simulink model "Modulary_loads"  (Simulink 8.1)
settings: Solver=ode23t  StartTime=0.0  StopTime=tfin  RelTol=1e-3
values from neighbouring files (symbols this model uses):
  C = 0    [Sketch_controller_model_ini.m]    (also in Symmetry_REAL_TIME_ini.m = 0.005; Symmetry_ini_Modulary.m = 0.02)
  C_ref = 20e-3    (= 0.02)    [Symmetry_ini_Modulary.m]
  IO = [1,1,1]    [Symmetry_ini_Modulary.m]
  main_IO = 1    [Symmetry_ini_Modulary.m]
  R = 100    [Sketch_controller_model_ini.m]    (also in Symmetry_REAL_TIME_ini.m; Symmetry_ini_Modulary.m = 50)
  R_ref = 50    [Symmetry_ini_Modulary.m]
  sample = 10e-5    (= 0.0001)    [Inverter_ini.m]    (also in Sketch_controller_model_ini.m; Symmetry_REAL_TIME_ini.m; Symmetry_ini.m; Symmetry_ini_COPY.m)
libraries: powerlib x17, powerlib_extras x3
settings Model: Creator=Neukirchner László  LastModifiedBy=Neukirchner László
settings SolverCC: ZeroCrossAlgorithm=Adaptive  SolverResetMethod=Robust
settings DataIOCC: SignalLoggingSaveFormat=Dataset
settings OptimizationCC: ExpressionDepthLimit=128
settings DebuggingCC: FcnCallInpInsideContextMsg=EnableAllAsError
settings GRTTargetCC: CombineOutputUpdateFcns=on  GRTInterface=off

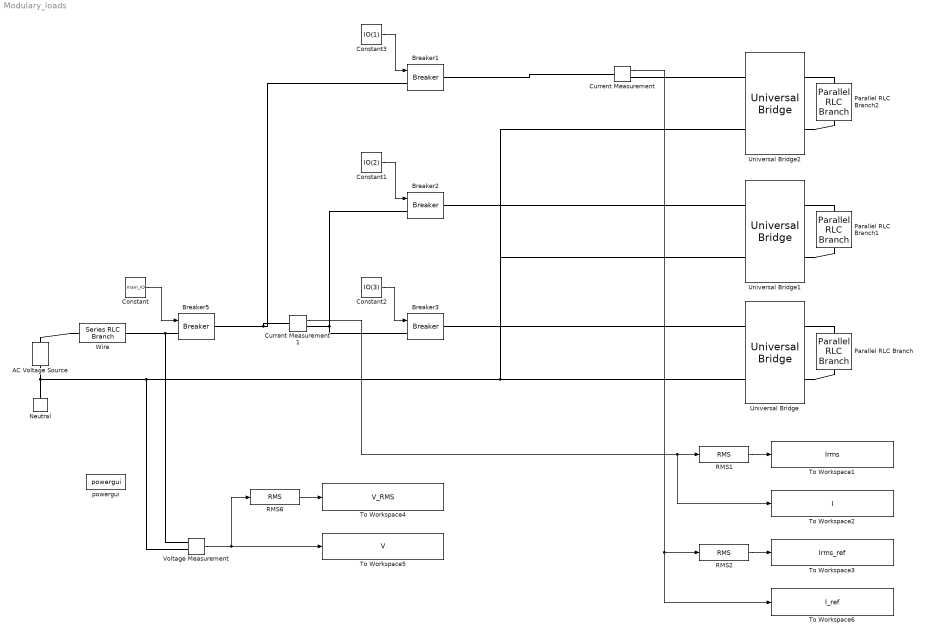
== system Modulary_loads ==
  AC Voltage Source : powerlib/Electrical Sources/AC Voltage Source  Amplitude=230*sqrt(2)  Phase=0  Frequency=50  SampleTime=sample  Measurements=None
  Breaker{1..3,5} (4 alike) : powerlib/Elements/Breaker  BreakerResistance=0.01  InitialState=0  SnubberResistance=1e7  SnubberCapacitance=inf  SwitchingTimes="[ 1/60  5/60 ]"  External=on  Measurements=None  MoreParameters=off  NoBreakLoop=off
  Constant : Constant  Value=main_IO
  Constant1 : Constant  Value=IO(2)
  Constant2 : Constant  Value=IO(3)
  Constant3 : Constant  Value=IO(1)
  Current Measurement : powerlib/Measurements/Current Measurement  PhasorSimulation=off  OutputType=Complex  PSBequivalent=0
  Current Measurement1 : powerlib/Measurements/Current Measurement  PhasorSimulation=off  OutputType=Complex  PSBequivalent=0
  Neutral : powerlib/Elements/Neutral  LConnTagsString=a  NodeNumber=10
  Parallel RLC Branch : powerlib/Elements/Parallel RLC Branch  LConnTagsString=a  RConnTagsString=__new0  BranchType=RC  Resistance=R  Inductance=1e-3  SetiL0=off  InitialCurrent=0  Capacitance=C  Setx0=off  InitialVoltage=0  Measurements=None
  Parallel RLC Branch1 : powerlib/Elements/Parallel RLC Branch  LConnTagsString=a  RConnTagsString=__new0  BranchType=RC  Resistance=R  Inductance=1e-3  SetiL0=off  InitialCurrent=0  Capacitance=C  Setx0=off  InitialVoltage=0  Measurements=None
  Parallel RLC Branch2 : powerlib/Elements/Parallel RLC Branch  LConnTagsString=a  RConnTagsString=__new0  BranchType=RC  Resistance=R_ref  Inductance=1e-3  SetiL0=off  InitialCurrent=0  Capacitance=C_ref  Setx0=off  InitialVoltage=0  Measurements=None
  RMS1 : powerlib_extras/Measurements/RMS  f1=50
  RMS2 : powerlib_extras/Measurements/RMS  f1=50
  RMS6 : powerlib_extras/Measurements/RMS  f1=50
  To Workspace1 : ToWorkspace  VariableName=Irms  SampleTime=sample  SaveFormat=Timeseries
  To Workspace2 : ToWorkspace  VariableName=I  SampleTime=sample  SaveFormat=Timeseries
  To Workspace3 : ToWorkspace  VariableName=Irms_ref  SampleTime=sample  SaveFormat=Timeseries
  To Workspace4 : ToWorkspace  VariableName=V_RMS  SampleTime=sample  SaveFormat=Timeseries
  To Workspace5 : ToWorkspace  VariableName=V  SampleTime=sample  SaveFormat=Timeseries
  To Workspace6 : ToWorkspace  VariableName=I_ref  SampleTime=sample  SaveFormat=Timeseries
  Universal Bridge : powerlib/Power Electronics/Universal Bridge  Arms=2  SnubberResistance=1e5  SnubberCapacitance=inf  Device=Diodes  Ron=1e-3  Lon=0  ForwardVoltages="[  0  0  ]"  ForwardVoltage=0.8  GTOparameters=[ 10e-6 , 20e-6 ]  IGBTparameters=[ 1e-6 , 2e-6 ]  Measurements=None  Measurements_2=None  converterType=Rectifier
  Universal Bridge1 : powerlib/Power Electronics/Universal Bridge  Arms=2  SnubberResistance=1e5  SnubberCapacitance=inf  Device=Diodes  Ron=1e-3  Lon=0  ForwardVoltages="[  0  0  ]"  ForwardVoltage=0.8  GTOparameters=[ 10e-6 , 20e-6 ]  IGBTparameters=[ 1e-6 , 2e-6 ]  Measurements=None  Measurements_2=None  converterType=Rectifier
  Universal Bridge2 : powerlib/Power Electronics/Universal Bridge  Arms=2  SnubberResistance=1e5  SnubberCapacitance=inf  Device=Diodes  Ron=1e-3  Lon=0  ForwardVoltages="[  0  0  ]"  ForwardVoltage=0.8  GTOparameters=[ 10e-6 , 20e-6 ]  IGBTparameters=[ 1e-6 , 2e-6 ]  Measurements=None  Measurements_2=None  converterType=Rectifier
  Voltage Measurement : powerlib/Measurements/Voltage Measurement  PhasorSimulation=off  OutputType=Complex  PSBequivalent=0
  Wire : powerlib/Elements/Series RLC Branch  LConnTagsString=__new0  RConnTagsString=__new0  BranchType=RL  Resistance=0.4  Inductance=1e-3  SetiL0=off  InitialCurrent=0  Capacitance=1e-6  Setx0=off  InitialVoltage=0  Measurements=None
  powergui : powerlib/powergui  SimulationMode=Continuous  SolverType=Tustin  SampleTime=50e-6  frequency=60  SPID=off  DisableSnubberDevices=off  DisableRonSwitches=off  DisableVfSwitches=off  SwTol=0  Interpol=off  DisplayEquations=off  frequencyindice=0  Pbase=100e6  ErrMax=1e-4  Iterations=50  UnitsV=kV  UnitsW=MW  FunctionMessages=off  echomessages=off  HookPort=off  EnableUseOfTLC=off  x0status=blocks  RestoreLinks=warning  ResistiveCurrentMeasurement=off  Frange=[0:2:500]  Ylog=off  Xlog=on  ShowGrid=off  save=off  variable=ZData  structure=0  ZoomFFT=on  StartTime=0.0  cycles=1  DisplayStyle=1  fundamental=60  FreqAxis=off  MaxFrequency=1000  frequencyindicesteady=1  RmsSteady=1  display=off  Ts=0  methode=off
  wires:
  RMS6/1 -> To Workspace4/1
  Constant/1 -> Breaker5/1
  Voltage Measurement/1 -> RMS6/1, To Workspace5/1
  Constant1/1 -> Breaker2/1
  Constant2/1 -> Breaker3/1
  Constant3/1 -> Breaker1/1
  RMS1/1 -> To Workspace1/1
  RMS2/1 -> To Workspace3/1
  Current Measurement1/1 -> To Workspace2/1, RMS1/1
  Current Measurement/1 -> To Workspace6/1, RMS2/1
  connections:
  Universal Bridge/LConn2 -- Voltage Measurement/LConn2 -- AC Voltage Source/LConn1 -- Neutral/LConn1 -- Universal Bridge2/LConn2 -- Universal Bridge1/LConn2
  Universal Bridge/RConn2 -- Parallel RLC Branch/RConn1
  Universal Bridge/RConn1 -- Parallel RLC Branch/LConn1
  Breaker5/LConn1 -- Voltage Measurement/LConn1 -- Wire/RConn1
  Wire/LConn1 -- AC Voltage Source/RConn1
  Universal Bridge1/RConn2 -- Parallel RLC Branch1/RConn1
  Universal Bridge1/RConn1 -- Parallel RLC Branch1/LConn1
  Breaker3/RConn1 -- Universal Bridge/LConn1
  Breaker1/LConn1 -- Current Measurement1/LConn1 -- Breaker5/RConn1
  Universal Bridge2/RConn1 -- Parallel RLC Branch2/LConn1
  Universal Bridge2/RConn2 -- Parallel RLC Branch2/RConn1
  Universal Bridge2/LConn1 -- Current Measurement/RConn1
  Current Measurement/LConn1 -- Breaker1/RConn1
  Breaker3/LConn1 -- Current Measurement1/RConn1 -- Breaker2/LConn1
  Universal Bridge1/LConn1 -- Breaker2/RConn1
